simulink model "Pressures"  (R2024b)
settings: Solver=VariableStepAuto  StartTime=0  StopTime=1500  RelTol=1e-3
libraries: simulink x2
settings Model: Creator=owen  LastModifiedBy=owen

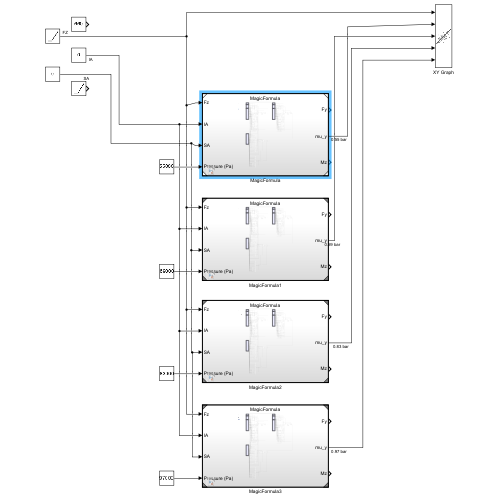
[thumbnail: Simulink's stored preview of the top-level diagram]
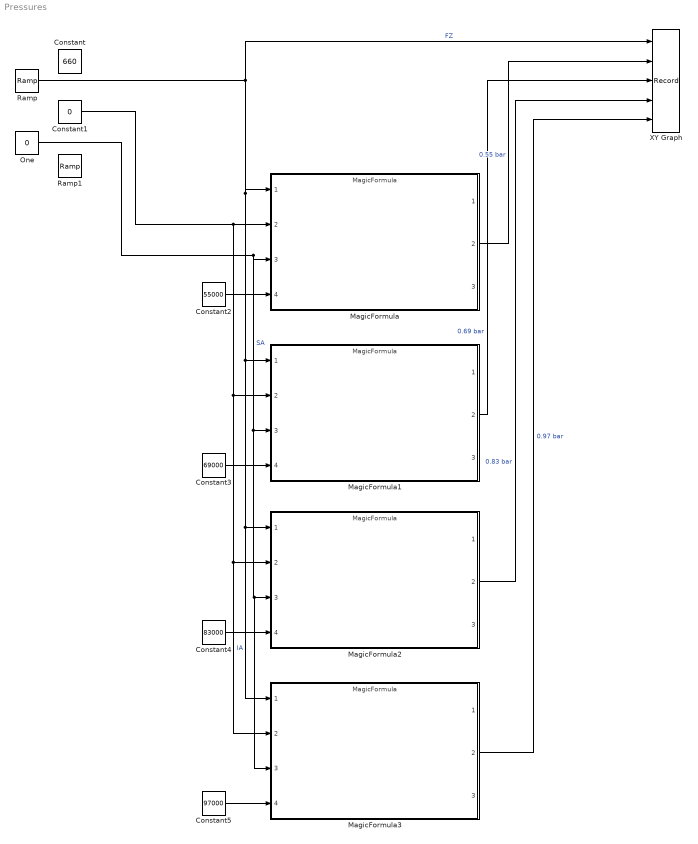
== system Pressures ==
  Constant : Constant  Value=660
  Constant1 : Constant  Value=0
  Constant2 : Constant  Value=55000
  Constant3 : Constant  Value=69000
  Constant4 : Constant  Value=83000
  Constant5 : Constant  Value=97000
  MagicFormula{,1..3} (4 alike) : ModelReference  ModelNameDialog=MagicFormula.slx  SimulationMode=Normal  ModelReferenceVersion=1.52
  One : Constant  Value=0  OutDataTypeStr=Inherit: Inherit via back propagation
  Ramp : simulink/Sources/Ramp  slope=1  start=0  InitialOutput=0
  Ramp1 : simulink/Sources/Ramp  slope=1  start=0  InitialOutput=-15
  XY Graph : Record  FileSettingsInternal="{\"entries\":[{\"content\":{\"excelSettings\":{\"content\":{},\"type\":\"Streamout.ExcelSettings\"}},\"type\":\"Streamout.FileSettingStorage\",\"uuid\":\"\"}],\"packageUris\":[\"http:\\/\\/schema.mathworks.com\\/mf0\\/streamout_blocks\\/R2020a\"],\"version\":\"1.0\"}"  Layout=[1 1]  SignalsInternal="{\"entries\":[{\"content\":{\"signals\":[{\"content\":{\"blockPath\":[],\"dimensions\":[1],\"domain\":\"\",\"lineColor\":\"#a2142f\",\"plots\":[ 1 ],\"port\":1,\"sid\":[\"\"],\"signalID\":1,\"signalName\":\"FZ\"},\"type\":\"RecordBlkView.Signal\",\"uuid\":\"\"},{\"content\":{\"blockPath\":[],\"dimensions\":[1],\"domain\":\"\",\"lineColor\":\"#139fff\",\"plots\":[ 1 ],\"port\":2,\"sid\":[\"\"],\"signalID\":2,\"signalName\":\"0.55 bar\"},\"type\":\"RecordBlkView.Signal\",\"uuid\":\"\"},{\"content\":{\"blockPath\":[],\"dimensions\":[1],\"domain\":\"\",\"lineColor\":\"#ff6929\",\"lineWidth\":2,\"plots\":[ 1 ],\"port\":3,\"sid\":[\"\"],\"signalID\":3,\"signalName\":\"0.69 bar\"},\"type\":\"RecordBlkView.Signal\",\"uuid\":\"\"},{\"content\":{\"blockPath\":[],\"dimensions\":[1],\"domain\":\"\",\"lineColor\":\"#b746ff\",\"lineWidth\":2,\"plots\":[ 1 ],\"port\":4,\"sid\":[\"\"],\"signalID\":4,\"signalName\":\"0.83 bar\"},\"type\":\"RecordBlkView.Signal\",\"uuid\":\"\"},{\"content\":{\"blockPath\":[],\"dimensions\":[1],\"domain\":\"\",\"lineColor\":\"#64d413\",\"lineWidth\":2,\"plots\":[ 1 ],\"port\":5,\"sid\":[\"\"],\"signalID\":5,\"signalName\":\"0.97 bar\"},\"type\":\"RecordBlkView.Signal\",\"uuid\":\"\"}]},\"type\":\"RecordBlkView.InputSignals\",\"uuid\":\"\"}],\"packageUris\":[\"http:\\/\\/schema.mathworks.com\\/mf0\\/streamout_blocks\\/R2020a\"],\"version\":\"1.0\"}"  VisualizationBindings="{\"xyplotplugin\":{\"info\":[{\"series\":[{\"bindingParametersList\":[{\"parameter\":\"X-Axis\",\"signalID\":1,\"signalName\":\"FZ\"},{\"parameter\":\"Y-Axis\",\"signalID\":2,\"signalName\":\"0.55 bar\"}],\"seriesID\":0},{\"bindingParametersList\":[{\"parameter\":\"X-Axis\",\"signalID\":1,\"signalName\":\"FZ\"},{\"parameter\":\"Y-Axis\",\"signalID\":3,\"signalName\":\"0.69 bar\"}],\"seriesID\":1},{\"bindingParametersList\":[{\"parameter\":\"X-Axis\",\"signalID\":1,\"signalName\":\"FZ\"},{\"parameter\":\"Y-Axis\",\"signalID\":4,\"signalName\":\"0.83 bar\"}],\"seriesID\":2},{\"bindingParametersList\":[{\"parameter\":\"X-Axis\",\"signalID\":1,\"signalName\":\"FZ\"},{\"parameter\":\"Y-Axis\",\"signalID\":5,\"signalName\":\"0.97 bar\"}],\"seriesID\":3}],\"subplotID\":1}]}}"  CompatibilityTag=XY
  wires:
  Ramp/1 -> MagicFormula3/1, MagicFormula2/1, MagicFormula1/1, MagicFormula/1, XY Graph/1  "FZ"
  One/1 -> MagicFormula3/3, MagicFormula2/3, MagicFormula1/3, MagicFormula/3  "SA"
  Constant1/1 -> MagicFormula3/2, MagicFormula2/2, MagicFormula1/2, MagicFormula/2  "IA"
  Constant2/1 -> MagicFormula/4
  MagicFormula/2 -> XY Graph/2  "0.55 bar"
  Constant3/1 -> MagicFormula1/4
  Constant5/1 -> MagicFormula3/4
  Constant4/1 -> MagicFormula2/4
  MagicFormula3/2 -> XY Graph/5  "0.97 bar"
  MagicFormula2/2 -> XY Graph/4  "0.83 bar"
  MagicFormula1/2 -> XY Graph/3  "0.69 bar"
